simulink model "rectificador_pwm_para_ver_curvas_igbt"  (R2024a)
settings: Solver=ode23t  StartTime=0.0  StopTime=2  FixedStep=sim_sample_time  MaxStep=1e-5  RelTol=1e-9
undefined symbols (not defined in the file or in its folder): config, gcbh, sps_rtmsupport, spsTwoLevelConverterModel, SwitchingDevices
libraries: spsIGBTDiodeLib x6, slpidlib x3, spsSeriesRLCBranchLib x2, spsabctodq0Lib x2, simulink x2, spsThreePhaseVIMeasurementLib x2, spsDCVoltageSourceLib x1, spsGroundLib x1, spsPLL3phLib x1, spsSVPWMGenerator2LevelLib x1, spsdq0toAlphaBetaZeroLib x1, spsdq0toabcLib x1
settings Model: SimulationMode=accelerator  PauseTimes=0.05  Creator=sebar  LastModifiedBy=sebar
settings SolverCC: ZeroCrossAlgorithm=Adaptive  AlgebraicLoopSolver=TrustRegion  DecoupledContinuousIntegration=on  ODENIntegrationMethod=ode14x
settings DataIOCC: ExternalInput=getinputstruct(op_trim1)  InitialState=steady_state  LimitDataPoints=on  LoadInitialState=on  SaveFinalState=on  SaveFormat=Array  SaveOutput=off  SignalLogging=off  DSMLogging=off  SaveTime=off
settings OptimizationCC: LifeSpan=inf
settings DebuggingCC: ReadBeforeWriteMsg=DisableAll  WriteAfterWriteMsg=DisableAll  WriteAfterReadMsg=DisableAll  IgnoredZcDiagnostic=none  SolverPrmCheckMsg=warning  MultiTaskDSMMsg=none  SFUnexpectedBacktrackingDiag=warning  SFNoUnconditionalDefaultTransitionDiag=warning  SFExecutionAtInitializationDiag=none  ArithmeticOperatorsInVariantConditions=warning
settings HardwareCC: ProdBitPerPointer=32  ProdBitPerSizeT=32  ProdBitPerPtrDiffT=32  ProdLargestAtomicFloat=None  ProdIntDivRoundTo=Undefined  ProdEndianess=Unspecified  ProdWordSize=32  ProdHWDeviceType=32-bit Generic
settings ModelReferenceCC: UpdateModelReferenceTargets=IfOutOfDate  PropagateSignalLabelsOutOfModel=off
settings SFSimCC: SFSimEcho=off  SimUseLocalCustomCode=off  CustomCodeUndefinedFunction=UseInterfaceOnly  SimTargetLang=C++  GPUAcceleration=on  SimDLTargetLibrary=cudnn
settings RTWCC: RTWUseLocalCustomCode=off  GPUComputeCapability=3.5
settings CodeAppCC: StateflowObjectComments=on
settings GRTTargetCC: TargetLangStandard=C89/C90 (ANSI)
settings ConfigComp: CovMetricSettings=dw  CovSaveCumulativeToWorkspaceVar=on  CovSaveSingleToWorkspaceVar=on  CovExternalEMLEnable=off  CovSFcnEnable=off
settings SimscapeCC: SimscapeNormalizeSystem=off

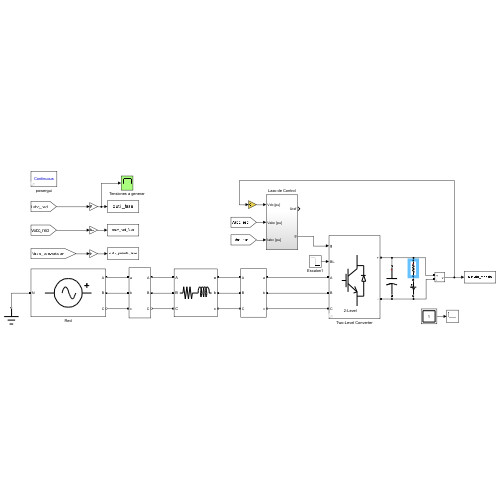
[thumbnail: Simulink's stored preview of the top-level diagram]
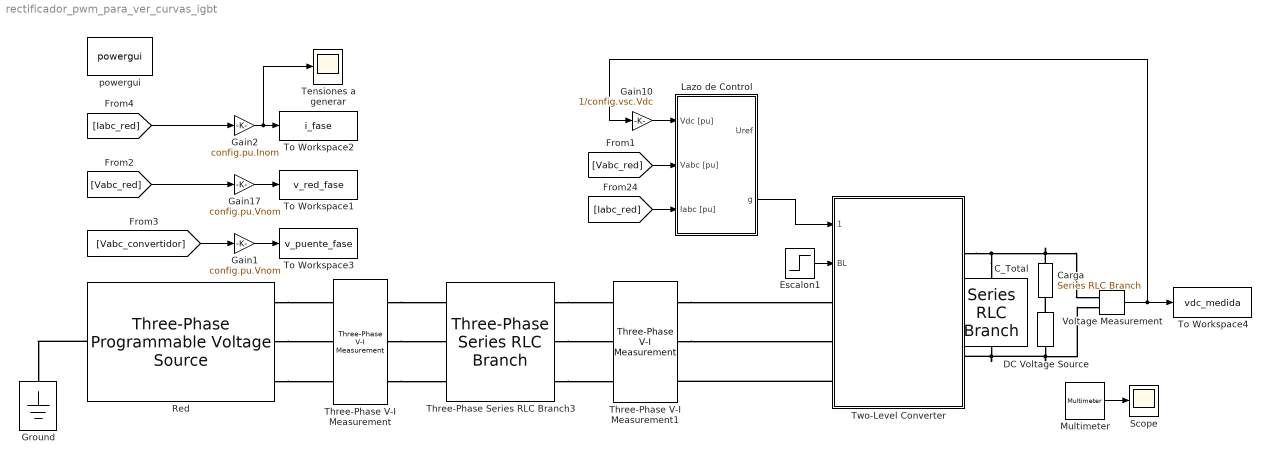
== system rectificador_pwm_para_ver_curvas_igbt ==
  C_Total : spsSeriesRLCBranchLib/Series RLC Branch  LConnTagsString=__new0  RConnTagsString=__new0  BranchType=C  Resistance=1  Inductance=1e-3  SetiL0=off  InitialCurrent=0  Capacitance=config.vsc.C  Setx0=on  InitialVoltage=config.vsc.Vdc  Measurements=Branch current
  Carga : spsSeriesRLCBranchLib/Series RLC Branch  LConnTagsString=__new0  RConnTagsString=__new0  BranchType=R  Resistance=config.vsc.R_load * ~config.usar_fuente_lado_DC + 1e-6 * config.usar_fuente_lado_DC  Inductance=1e-3  SetiL0=off  InitialCurrent=0  Capacitance=1e-6  Setx0=off  InitialVoltage=0  Measurements=None
  DC Voltage Source : spsDCVoltageSourceLib/DC Voltage Source  Amplitude=config.vsc.Vdc * config.usar_fuente_lado_DC  Measurements=None
  Escalon1 : Step  Time=0.25*(config.mode == ModoControl.SOLO_FEEDFORWARD)*0  Before=1  After=0  SampleTime=1e-5
  Gain1 : Gain  Gain=config.pu.Vnom
  Gain10 : Gain  Gain=1/config.vsc.Vdc
  Gain17 : Gain  Gain=config.pu.Vnom
  Gain2 : Gain  Gain=config.pu.Inom
  Ground : spsGroundLib/Ground  LConnTagsString=a
  Lazo de Control : Subsystem
  Multimeter : spsMultimeterLib/Multimeter  L=1  sel=1  yselected={}  Gain=1  OutputType=Complex  PlotAtSimulationStop=off  PhasorSimulation=off
  Red : spsThreePhaseProgrammableVoltageSourceLib/Three-Phase Programmable Voltage Source  PositiveSequence="[28*sqrt(3)  0 50]"  VariationEntity=None  VariationType=Step  VariationTypeAlt=Step  VariationStep=1  VariationRate=10  VariationMagnitude=0.3  VariationFrequency=2  VariationTiming=[1 2]  VariationPhaseA=off  Amplitudes=[1 0.8 1.2 1.0]  TimeValues=[0 0.1 0.15 0.2]  HarmonicGeneration=off  HarmonicA=[3 0.2 -25 0]  HarmonicB=[2 0.15 35 2]  Timing="[0.05  3]"  BusType=swing  Pref=0  Qref=0  Qmin=-inf  Qmax=inf
  Scope : Scope
  Tensiones a generar : Scope
  Three-Phase Series RLC Branch3 : spsThreePhaseSeriesRLCBranchLib/Three-Phase Series RLC Branch  LConnTagsString=A|B|C  RConnTagsString=A|B|C  BranchType=RL  Resistance=config.vsc.R  Inductance=config.vsc.L  Capacitance=1e-6  Measurements=None
  Three-Phase V-I Measurement : spsThreePhaseVIMeasurementLib/Three-Phase V-I Measurement  VoltageMeasurement=phase-to-ground  SetLabelV=on  LabelV=Vabc_red  Vpu=on  VpuLL=off  CurrentMeasurement=yes  SetLabelI=on  LabelI=Iabc_red  Ipu=on  Pbase=config.pu.Pnom  Vbase=config.pu.Vnom * sqrt(3) / sqrt(2)  OutputType=Complex  PhasorSimulation=off  PSBequivalent=0
  Three-Phase V-I Measurement1 : spsThreePhaseVIMeasurementLib/Three-Phase V-I Measurement  VoltageMeasurement=phase-to-ground  SetLabelV=on  LabelV=Vabc_convertidor  Vpu=on  VpuLL=off  CurrentMeasurement=no  SetLabelI=off  LabelI=Iabc  Ipu=off  Pbase=100e6  Vbase=config.pu.Vnom * sqrt(3) / sqrt(2)  OutputType=Complex  PhasorSimulation=off  PSBequivalent=0
  To Workspace1 : ToWorkspace  VariableName=v_red_fase  SaveFormat=Timeseries  SampleTime=config.to_workspace_sample_time
  To Workspace2 : ToWorkspace  VariableName=i_fase  SaveFormat=Timeseries  SampleTime=config.to_workspace_sample_time
  To Workspace3 : ToWorkspace  VariableName=v_puente_fase  SaveFormat=Timeseries  SampleTime=config.to_workspace_sample_time
  To Workspace4 : ToWorkspace  VariableName=vdc_medida  SaveFormat=Timeseries  SampleTime=config.to_workspace_sample_time
  Two-Level Converter : Subsystem  AncestorBlock=sps_lib/Power Electronics/Two-Level Converter  DialogController=POWERSYS.PowerSysDialog  LoadFcn=sps_rtmsupport('LoadFcn',gcbh);  StartFcn=sps_rtmsupport('StartFcn',gcbh);  StopFcn=sps_rtmsupport('StopFcn',gcbh);  mask(Two-Level Converter){ModelType=Switching devices, Ron=1e-6, Rs=config.vsc.snubber.Rs, Cs=config.vsc.snubber.Cs, Vforward=[0,0], Ron_Diode=1e-3, Rs_Diode=1e6, Cs_Diode=inf, Vf_Diode=1e-3, Rs_CurrentSource=inf, Ron_ACsource=1e-3}
      mask prompts: ModelType "Model type:"; Ron "Device on-state resistance (Ohms)"; Rs "Snubber resistance (Ohms)"; Cs "Snubber capacitance (F)"; Vforward "Forward voltages [Device Vf(V), Diode Vfd(V)]"; Ron_Diode "Diode on-state resistance (Ohms)"; Rs_Diode "Diode snubber resistance (Ohms)"; Cs_Diode "Diode snubber capacitance (F)"; Vf_Diode "Diode forward voltage (V)"; Rs_CurrentSource "DC side snubber resistance (Ohms)"; Ron_ACsource "AC side source resistance (Ohms)"
      mask help:
      | Implements a three-phase two-level power converter using the following modeling techniques:
      |
      | 1. Switching devices: The converter is modeled with IGBT/diode pairs controlled by firing pulses produced by a PWM generator.
      |
      | 2. Switching function: The converter is modeled by a switching function controlled by firing pulses produced by a PWM generator (0/1 signals) or by firing pulses averaged over a specified period (PWM averaging: signals between 0 and 1).
      |
      | 3. Average model (Uref-controlled): The converter is modeled using a switching-function model directly controlled by the reference voltage. A PWM generator is not required.
      |
      | 4. Average model (Uref-controlled, no rectifier mode): The converter is modeled using voltage sources directly controlled by the reference voltage. A PWM generator is not required, and the rectifier mode is not simulated.
      |
      | Technique 1 is the most accurate, while technique 4 yields to the fastest simulation. Technique 2 (with firing pulses averaged), as well as techniques 3 and 4 are well-suited for real-time simulation.
      mask init:
      | block=gcb;
      | [WantBlockChoice,Ts,BLK] = powericon('PowerConverterCback',block,Ron,Rs,Cs,Vforward,Ron_Diode,Rs_Diode,Cs_Diode,Vf_Diode,Rs_CurrentSource, Ron_ACsource);
      | powericon('SetInternalModels','set',block,WantBlockChoice);
      settings: LibrarySourceBlock=sps_lib/Power Electronics/Two-Level Converter  CopyFcn=sps_rtmsupport('CopyFcn',gcbh);  DeleteFcn=sps_rtmsupport('DeleteFcn',gcbh);  UndoDeleteFcn=sps_rtmsupport('UndoDeleteFcn',gcbh);  ModelCloseFcn=sps_rtmsupport('ModelCloseFcn',gcbh);  PreSaveFcn=sps_rtmsupport('PreSaveFcn',gcbh);  PostSaveFcn=sps_rtmsupport('PostSaveFcn',gcbh);  NameChangeFcn=sps_rtmsupport('NameChangeFcn',gcbh);  PreCopyFcn=sps_rtmsupport('PreCopyFcn',gcbh);  OpenFcn=sps_rtmsupport('OpenFcn',gcbh, [1]);  CloseFcn=sps_rtmsupport('CloseFcn',gcbh);  PreDeleteFcn=sps_rtmsupport('PreDeleteFcn',gcbh);
      mask Help: helpview(psbhelp);
      mask TypeOptions ModelType: Switching devices | Switching function | Average model (Uref-controlled) | Average model (No rectifier mode)
      mask Callback ModelType: powericon('PowerConverterCback',gcb);
      mask Display:
      | x1=0.05;
      | y1=0.20;
      | %
      | plot([0.5 0.5]+x1,[0.97,0.8]-y1)
      | plot([0.5 0.32]+x1,[0.80 0.71]-y1)
      | plot([0.32 0.32]+x1,[0.80 0.52]-y1)
      | plot([0.32 0.5]+x1,[0.62 0.52]-y1)
      | plot([0.5 0.5]+x1,[0.52 0.35]-y1)
      | plot([0.45 0.5 0.43]+x1,[0.59 0.52 0.51]-y1)
      | %
      | plot([0.28 0.28]+x1,[0.74 0.58]-y1)
      | plot([0.28 0.20]+x1,[0.66 0.66]-y1)
      | %
      | plot([0.5 0.63]+x1,[0.84 0.84]-y1)
      | plot([0.63 0.63]+x1,[0.84 0.72]-y1)
      | plot([0.63 0.59]+x1,[0.72 0.65]-y1)
      | plot([0.63 0.67]+x1,[0.72 0.65]-y1)
      | plot([0.59 0.67]+x1,[0.65 0.65]-y1)
      | plot([0.63 0.63]+x1,[0.65 0.47]-y1)
      | plot([0.5 0.63]+x1,[0.47 0.47]-y1)
      | plot([0.58 0.67]+x1,[0.72 0.72]-y1)
      | %
      | text(0.3,0.1,'2-Level')
      | if ModelType==3 |ModelType==4
      |    port_label('input',1,'Uref')
      | else
      |     port_label('input',1,'g')
      | end
  Voltage Measurement : spsVoltageMeasurementLib/Voltage Measurement  PhasorSimulation=off  OutputType=Complex  PSBequivalent=0
  powergui : sps_lib/powergui  Priority=1  SimulationMode=Continuous  SampleTime=config.sample_time  frequency=50  Iterations=50  frequencyindice=0  Pbase=100e6  ErrMax=1e-4  UnitsV=kV  UnitsW=MW  buscounter=0  FunctionMessages=off  echomessages=off  EnableUseOfTLC=off  CurrentSourceSwitches=on  DisableSnubberDevices=off  DisableRonSwitches=off  DisableVfSwitches=off  DisplayEquations=off  AutomaticDiscreteSolvers=off  SolverType=Tustin  Interpol=off  ExternalGateDelay=off  methode=on  Ts=100  x0status=blocks  SPID=off  SwTol=0  HookPort=off  NonlinearTolerance=1e-4  nMaxIteration=100  ContinueOnMaxIteration=off  RestoreLinks=warning  ResistiveCurrentMeasurement=off  Frange=[0:2:500]  Ylog=off  Xlog=on  ShowGrid=off  save=off  variable=ZData  structure=0  ZoomFFT=off  StartTime=0.0  cycles=1  DisplayStyle=1  fundamental=60  FreqAxis=off  MaxFrequency=1000  frequencyindicesteady=1  RmsSteady=1  display=off
  wires:
  Gain10/1 -> Lazo de Control/1(Vdc [pu])
  [Vabc_red] -> Lazo de Control/2(Vabc [pu])
  [Iabc_red] -> Lazo de Control/3(Iabc [pu])
  [Vabc_convertidor] -> Gain1/1
  [Vabc_red] -> Gain17/1
  Voltage Measurement/1 -> Gain10/1, To Workspace4/1
  Gain17/1 -> To Workspace1/1
  Gain1/1 -> To Workspace3/1
  Escalon1/1 -> Two-Level Converter/2(BL)
  Gain2/1 -> Tensiones a generar/1, To Workspace2/1
  [Iabc_red] -> Gain2/1
  Lazo de Control/2(g) -> Two-Level Converter/1("  ")
  Multimeter/1 -> Scope/1
  connections:
  Red/LConn1 -- Ground/LConn1
  C_Total/RConn1 -- DC Voltage Source/LConn1 -- Voltage Measurement/LConn2 -- Two-Level Converter/RConn2
  C_Total/LConn1 -- Carga/LConn1 -- Voltage Measurement/LConn1 -- Two-Level Converter/RConn1
  Three-Phase Series RLC Branch3/RConn1 -- Three-Phase V-I Measurement1/LConn1
  Three-Phase Series RLC Branch3/RConn2 -- Three-Phase V-I Measurement1/LConn2
  Three-Phase Series RLC Branch3/RConn3 -- Three-Phase V-I Measurement1/LConn3
  Three-Phase V-I Measurement1/RConn1 -- Two-Level Converter/LConn1
  Three-Phase V-I Measurement1/RConn2 -- Two-Level Converter/LConn2
  Two-Level Converter/LConn3 -- Three-Phase V-I Measurement1/RConn3
  Three-Phase V-I Measurement/LConn1 -- Three-Phase Series RLC Branch3/LConn1
  Three-Phase V-I Measurement/LConn2 -- Three-Phase Series RLC Branch3/LConn2
  Three-Phase V-I Measurement/LConn3 -- Three-Phase Series RLC Branch3/LConn3
  Red/RConn1 -- Three-Phase V-I Measurement/RConn1
  Red/RConn2 -- Three-Phase V-I Measurement/RConn2
  Red/RConn3 -- Three-Phase V-I Measurement/RConn3
  DC Voltage Source/RConn1 -- Carga/RConn1

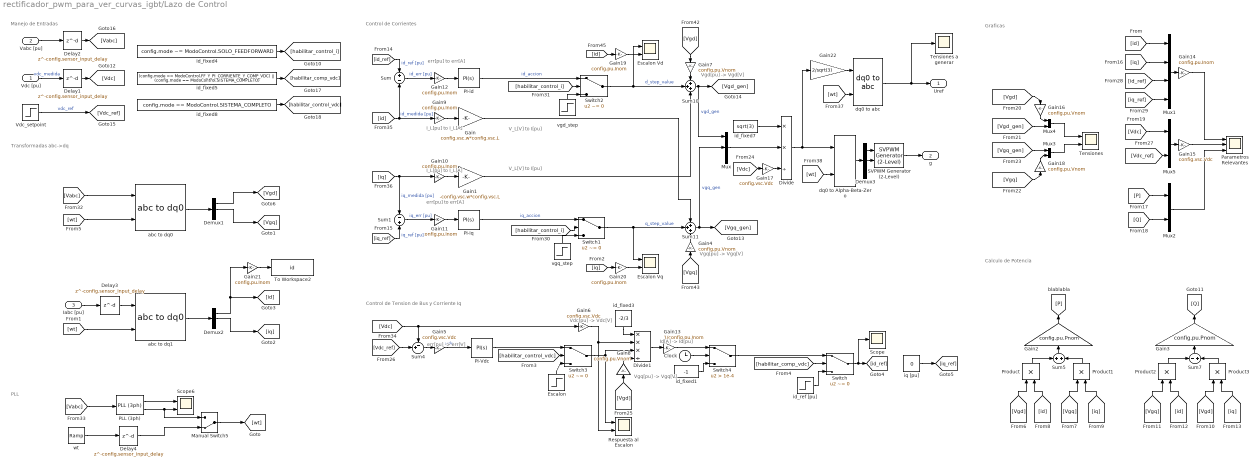
== system rectificador_pwm_para_ver_curvas_igbt/Lazo de Control ==
  note: Transformadas abc->dq
  note: I_L[pu] to I_L[A]
  note: Calculo de Potencia
  note: Graficas
  note: PLL
  note: Manejo de Entradas
  note: Control de Tension de Bus y Corriente Iq
  note: Control de Corrientes
  note: V_L[V] to I[pu]
  note: Vgd[pu] -> Vgd[V]
  note: I_L[pu] to I_L[A]
  note: Vgq[pu] -> Vgq[V]
  note: Vgq[pu] -> Vgq[V]
  note: Id[A] -> Id[pu]
  note: err[pu] -> err[V]
  note: err[pu] to err[A]
  note: err[pu] to err[A]
  note: Vdc[pu] -> Vdc[V]
  note: V_L[V] to I[pu]
  Vdc [pu] : Inport
  Vabc [pu] : Inport  Port=2
  Iabc [pu] : Inport  Port=3
  Clock : Clock
  Delay1 : Delay  DelayLength=config.sensor_input_delay  InitialCondition=1  SampleTime=config.sensor_input_sample_time
  Delay2 : Delay  DelayLength=config.sensor_input_delay  InitialCondition=1  SampleTime=config.sensor_input_sample_time
  Delay3 : Delay  DelayLength=config.sensor_input_delay  InitialCondition=1  SampleTime=config.sensor_input_sample_time
  Delay4 : Delay  DelayLength=config.sensor_input_delay  InitialCondition=0  SampleTime=config.sensor_input_sample_time
  Demux1 : Demux  Outputs=3
  Demux2 : Demux  Outputs=3
  Demux3 : Demux  Outputs=3
  Divide : Product  Inputs=**/
  Divide1 : Product  Inputs=***/
  Escalon : Step  Time=config.step.id.time  Before=config.step.id.start_value  After=config.step.id.end_value  SampleTime=1e-5
  Escalon Vd : Scope  NumInputPorts=2
  Escalon Vq : Scope  NumInputPorts=2
  Gain : Gain  Gain=config.vsc.w*config.vsc.L
  Gain1 : Gain  Gain=-config.vsc.w*config.vsc.L
  Gain{9..12,14,19..21} (8 alike) : Gain  Gain=config.pu.Inom
  Gain13 : Gain  Gain=1/config.pu.Inom
  Gain{5..6,15,17} (4 alike) : Gain  Gain=config.vsc.Vdc
  Gain{4,7..8,16,18} (5 alike) : Gain  Gain=config.pu.Vnom
  Gain2 : Gain  Gain=config.pu.Pnom
  Gain22 : Gain  Gain=2/sqrt(3)
  Gain3 : Gain  Gain=config.pu.Pnom
  Manual Switch5 : ManualSwitch  CurrentSetting=0
  Mux : Mux  Inputs=3
  Mux1 : Mux
  Mux{2..5} (4 alike) : Mux  Inputs=2
  PI-Vdc : slpidlib/PID Controller  Controller=PI  Form=Parallel  TimeDomain=Continuous-time  UseExternalTs=off  SampleTime=1  IntegratorMethod=Forward Euler  FilterMethod=Forward Euler  ControllerParametersSource=internal  P=config.ContDC.Kp  I=config.ContDC.Ki  UseKiTs=off  D=0  UseExternalDerivativeSource=off  N=100  UseFilter=on  TunerSelectOption=Transfer Function Based (PID Tuner App)  InitialConditionSource=internal  InitialConditionForIntegrator=0  InitialConditionForFilter=0  DifferentiatorICPrevScaledInput=0  ExternalReset=none  TrackingMode=off  Kt=1  LimitOutput=off  SatLimitsSource=internal  UpperSaturationLimit=inf  LowerSaturationLimit=-inf  LinearizeAsGain=on  AntiWindupMode=none  Kb=1  LimitIntegrator=off  UpperIntegratorSaturationLimit=inf  LowerIntegratorSaturationLimit=-inf  POutMin=[]  POutMax=[]  IOutMin=[]  IOutMax=[]  DOutMin=[]  DOutMax=[]  NOutMin=[]  NOutMax=[]  SumOutMin=[]  SumOutMax=[]  SaturationOutMin=[]  SaturationOutMax=[]  PParamMin=[]  PParamMax=[]  IParamMin=[]  IParamMax=[]  DParamMin=[]  DParamMax=[]  NParamMin=[]  NParamMax=[]  KbParamMin=[]  KbParamMax=[]  KtParamMin=[]  KtParamMax=[]  KbOutMin=[]  KbOutMax=[]  KtOutMin=[]  KtOutMax=[]  IntegratorOutMin=[]  IntegratorOutMax=[]  FilterOutMin=[]  FilterOutMax=[]  SumI1OutMin=[]  SumI1OutMax=[]  SumI2OutMin=[]  SumI2OutMax=[]  SumI3OutMin=[]  SumI3OutMax=[]  SumI4OutMin=[]  SumI4OutMax=[]  SumDOutMin=[]  SumDOutMax=[]  DifferentiatorOutMin=[]  DifferentiatorOutMax=[]  FilterDiffOutCoefMin=[]  FilterDiffOutCoefMax=[]  ReciprocalOutMin=[]  ReciprocalOutMax=[]  SumDenOutMin=[]  SumDenOutMax=[]  SumNumOutMin=[]  SumNumOutMax=[]  DivideOutMin=[]  DivideOutMax=[]  UdiffTsProdOutMin=[]  UdiffTsProdOutMax=[]  NTsProdOutMin=[]  NTsProdOutMax=[]  UintegralTsProdOutMin=[]  UintegralTsProdOutMax=[]  UngainTsProdOutMin=[]  UngainTsProdOutMax=[]  ClampingZeroOutDataTypeStr=Inherit: Inherit via back propagation  ClampingZeroOutMin=[]  ClampingZeroOutMax=[]  FilterDenConstantOutDataTypeStr=Inherit: Inherit via back propagation  FilterDenConstantOutMin=[]  FilterDenConstantOutMax=[]  PCopyOutDataTypeStr=Inherit: Inherit via back propagation  PCopyOutMin=[]  PCopyOutMax=[]  NCopyOutDataTypeStr=Inherit: Inherit via back propagation  NCopyOutMin=[]  NCopyOutMax=[]  IntegratorContinuousStateAttributes=''  IntegratorStateMustResolveToSignalObject=off  IntegratorRTWStateStorageClass=Auto  FilterContinuousStateAttributes=''  FilterStateMustResolveToSignalObject=off  FilterRTWStateStorageClass=Auto  ParallelPVariant=InternalParameters  IdealPVariant=Disabled  IVariant=InternalParameters  DVariant=Disabled  IntegratorVariant=Continuous  SatVariant=Disabled  AWVariant=Passthrough  PCopyVariant=Disabled  TRVariant=Disabled  FdbkBlocksVariant=Forward  IdealPFdbkVariant=Disabled  SatFdbkVariant=Disabled  DerivativeFilterVariant=Disabled  NVariant=Disabled  NCopyVariant=Disabled_SignalSpec  FilterICVariant=Disabled  IntegratorICVariant=InternalICs  ExternalResetVariant=Disabled  TRSumVariant=Passthrough  SumFdbkVariant=Disabled  SumVariant=Sum_PI  TsampFilterVariant=InternalTs  TsampNgainVariant=Passthrough  TsampIntegralVariant=Disabled_SignalSpec  ExternalSaturationOutDataTypeStr=Inherit: Same as second input  DerivativeSourceVariant=Disabled
  PI-id : slpidlib/PID Controller  Controller=PI  Form=Parallel  TimeDomain=Continuous-time  UseExternalTs=off  SampleTime=1  IntegratorMethod=Forward Euler  FilterMethod=Forward Euler  ControllerParametersSource=internal  P=config.ContI.Kp  I=config.ContI.Ki  UseKiTs=off  D=0  UseExternalDerivativeSource=off  N=100  UseFilter=on  TunerSelectOption=Transfer Function Based (PID Tuner App)  InitialConditionSource=internal  InitialConditionForIntegrator=0  InitialConditionForFilter=0  DifferentiatorICPrevScaledInput=0  ExternalReset=none  TrackingMode=off  Kt=1  LimitOutput=off  SatLimitsSource=internal  UpperSaturationLimit=20  LowerSaturationLimit=-20  LinearizeAsGain=on  AntiWindupMode=none  Kb=1  LimitIntegrator=off  UpperIntegratorSaturationLimit=inf  LowerIntegratorSaturationLimit=-inf  POutMin=[]  POutMax=[]  IOutMin=[]  IOutMax=[]  DOutMin=[]  DOutMax=[]  NOutMin=[]  NOutMax=[]  SumOutMin=[]  SumOutMax=[]  SaturationOutMin=[]  SaturationOutMax=[]  PParamMin=[]  PParamMax=[]  IParamMin=[]  IParamMax=[]  DParamMin=[]  DParamMax=[]  NParamMin=[]  NParamMax=[]  KbParamMin=[]  KbParamMax=[]  KtParamMin=[]  KtParamMax=[]  KbOutMin=[]  KbOutMax=[]  KtOutMin=[]  KtOutMax=[]  IntegratorOutMin=[]  IntegratorOutMax=[]  FilterOutMin=[]  FilterOutMax=[]  SumI1OutMin=[]  SumI1OutMax=[]  SumI2OutMin=[]  SumI2OutMax=[]  SumI3OutMin=[]  SumI3OutMax=[]  SumI4OutMin=[]  SumI4OutMax=[]  SumDOutMin=[]  SumDOutMax=[]  DifferentiatorOutMin=[]  DifferentiatorOutMax=[]  FilterDiffOutCoefMin=[]  FilterDiffOutCoefMax=[]  ReciprocalOutMin=[]  ReciprocalOutMax=[]  SumDenOutMin=[]  SumDenOutMax=[]  SumNumOutMin=[]  SumNumOutMax=[]  DivideOutMin=[]  DivideOutMax=[]  UdiffTsProdOutMin=[]  UdiffTsProdOutMax=[]  NTsProdOutMin=[]  NTsProdOutMax=[]  UintegralTsProdOutMin=[]  UintegralTsProdOutMax=[]  UngainTsProdOutMin=[]  UngainTsProdOutMax=[]  ClampingZeroOutDataTypeStr=Inherit: Inherit via back propagation  ClampingZeroOutMin=[]  ClampingZeroOutMax=[]  FilterDenConstantOutDataTypeStr=Inherit: Inherit via back propagation  FilterDenConstantOutMin=[]  FilterDenConstantOutMax=[]  PCopyOutDataTypeStr=Inherit: Inherit via back propagation  PCopyOutMin=[]  PCopyOutMax=[]  NCopyOutDataTypeStr=Inherit: Inherit via back propagation  NCopyOutMin=[]  NCopyOutMax=[]  IntegratorContinuousStateAttributes=''  IntegratorStateMustResolveToSignalObject=off  IntegratorRTWStateStorageClass=Auto  FilterContinuousStateAttributes=''  FilterStateMustResolveToSignalObject=off  FilterRTWStateStorageClass=Auto  ParallelPVariant=InternalParameters  IdealPVariant=Disabled  IVariant=InternalParameters  DVariant=Disabled  IntegratorVariant=Continuous  SatVariant=Disabled  AWVariant=Passthrough  PCopyVariant=Disabled  TRVariant=Disabled  FdbkBlocksVariant=Forward  IdealPFdbkVariant=Disabled  SatFdbkVariant=Disabled  DerivativeFilterVariant=Disabled  NVariant=Disabled  NCopyVariant=Disabled_SignalSpec  FilterICVariant=Disabled  IntegratorICVariant=InternalICs  ExternalResetVariant=Disabled  TRSumVariant=Passthrough  SumFdbkVariant=Disabled  SumVariant=Sum_PI  TsampFilterVariant=InternalTs  TsampNgainVariant=Passthrough  TsampIntegralVariant=Disabled_SignalSpec  ExternalSaturationOutDataTypeStr=Inherit: Same as second input  DerivativeSourceVariant=Disabled
  PI-iq : slpidlib/PID Controller  Controller=PI  Form=Parallel  TimeDomain=Continuous-time  UseExternalTs=off  SampleTime=1  IntegratorMethod=Forward Euler  FilterMethod=Forward Euler  ControllerParametersSource=internal  P=config.ContI.Kp  I=config.ContI.Ki  UseKiTs=off  D=0  UseExternalDerivativeSource=off  N=100  UseFilter=on  TunerSelectOption=Transfer Function Based (PID Tuner App)  InitialConditionSource=internal  InitialConditionForIntegrator=0  InitialConditionForFilter=0  DifferentiatorICPrevScaledInput=0  ExternalReset=none  TrackingMode=off  Kt=1  LimitOutput=off  SatLimitsSource=internal  UpperSaturationLimit=20  LowerSaturationLimit=-20  LinearizeAsGain=on  AntiWindupMode=none  Kb=1  LimitIntegrator=off  UpperIntegratorSaturationLimit=inf  LowerIntegratorSaturationLimit=-inf  POutMin=[]  POutMax=[]  IOutMin=[]  IOutMax=[]  DOutMin=[]  DOutMax=[]  NOutMin=[]  NOutMax=[]  SumOutMin=[]  SumOutMax=[]  SaturationOutMin=[]  SaturationOutMax=[]  PParamMin=[]  PParamMax=[]  IParamMin=[]  IParamMax=[]  DParamMin=[]  DParamMax=[]  NParamMin=[]  NParamMax=[]  KbParamMin=[]  KbParamMax=[]  KtParamMin=[]  KtParamMax=[]  KbOutMin=[]  KbOutMax=[]  KtOutMin=[]  KtOutMax=[]  IntegratorOutMin=[]  IntegratorOutMax=[]  FilterOutMin=[]  FilterOutMax=[]  SumI1OutMin=[]  SumI1OutMax=[]  SumI2OutMin=[]  SumI2OutMax=[]  SumI3OutMin=[]  SumI3OutMax=[]  SumI4OutMin=[]  SumI4OutMax=[]  SumDOutMin=[]  SumDOutMax=[]  DifferentiatorOutMin=[]  DifferentiatorOutMax=[]  FilterDiffOutCoefMin=[]  FilterDiffOutCoefMax=[]  ReciprocalOutMin=[]  ReciprocalOutMax=[]  SumDenOutMin=[]  SumDenOutMax=[]  SumNumOutMin=[]  SumNumOutMax=[]  DivideOutMin=[]  DivideOutMax=[]  UdiffTsProdOutMin=[]  UdiffTsProdOutMax=[]  NTsProdOutMin=[]  NTsProdOutMax=[]  UintegralTsProdOutMin=[]  UintegralTsProdOutMax=[]  UngainTsProdOutMin=[]  UngainTsProdOutMax=[]  ClampingZeroOutDataTypeStr=Inherit: Inherit via back propagation  ClampingZeroOutMin=[]  ClampingZeroOutMax=[]  FilterDenConstantOutDataTypeStr=Inherit: Inherit via back propagation  FilterDenConstantOutMin=[]  FilterDenConstantOutMax=[]  PCopyOutDataTypeStr=Inherit: Inherit via back propagation  PCopyOutMin=[]  PCopyOutMax=[]  NCopyOutDataTypeStr=Inherit: Inherit via back propagation  NCopyOutMin=[]  NCopyOutMax=[]  IntegratorContinuousStateAttributes=''  IntegratorStateMustResolveToSignalObject=off  IntegratorRTWStateStorageClass=Auto  FilterContinuousStateAttributes=''  FilterStateMustResolveToSignalObject=off  FilterRTWStateStorageClass=Auto  ParallelPVariant=InternalParameters  IdealPVariant=Disabled  IVariant=InternalParameters  DVariant=Disabled  IntegratorVariant=Continuous  SatVariant=Disabled  AWVariant=Passthrough  PCopyVariant=Disabled  TRVariant=Disabled  FdbkBlocksVariant=Forward  IdealPFdbkVariant=Disabled  SatFdbkVariant=Disabled  DerivativeFilterVariant=Disabled  NVariant=Disabled  NCopyVariant=Disabled_SignalSpec  FilterICVariant=Disabled  IntegratorICVariant=InternalICs  ExternalResetVariant=Disabled  TRSumVariant=Passthrough  SumFdbkVariant=Disabled  SumVariant=Sum_PI  TsampFilterVariant=InternalTs  TsampNgainVariant=Passthrough  TsampIntegralVariant=Disabled_SignalSpec  ExternalSaturationOutDataTypeStr=Inherit: Same as second input  DerivativeSourceVariant=Disabled
  PLL (3ph) : spsPLL3phLib/PLL (3ph)  Fmin=45  Par_Init=[0, config.vsc.f]  ParK=[180, 3200, 1]  TcD=1e-4  MaxRateChangeFreq=12  FilterCutOffFreq=25  Ts=1 / config.vsc.f_sw  AGC=on
  Parametros Relevantes : Scope  NumInputPorts=3
  Product{,1..3} (4 alike) : Product
  Respuesta al Escalon : Scope  NumInputPorts=2
  SVPWM Generator (2-Level) : spsSVPWMGenerator2LevelLib/SVPWM Generator (2-Level)  InputType=alpha-beta components  SwitchingPattern=Pattern #1  Fc=config.vsc.f_sw  ParUref=[0.8 -30 50]  Ts=1/config.vsc.f_sw*0
  Scope : Scope
  Scope6 : Scope  NumInputPorts=2
  Sum : Sum  Inputs=+|-
  Sum1 : Sum  Inputs=-|+
  Sum10 : Sum  Inputs=+++
  Sum11 : Sum  Inputs=+++
  Sum4 : Sum  Inputs=-+|
  Sum5 : Sum  Inputs=+|+
  Sum7 : Sum  Inputs=-|+
  Switch{,1..3} (4 alike) : Switch  Criteria=u2 ~= 0  SaturateOnIntegerOverflow=off  InputSameDT=off
  Switch4 : Switch  Criteria=u2 > Threshold  Threshold=1e-4  SaturateOnIntegerOverflow=off  InputSameDT=off
  Tensiones : Scope  NumInputPorts=2
  Tensiones a generar : Scope
  To Workspace2 : ToWorkspace  VariableName=id  SaveFormat=Timeseries  SampleTime=config.to_workspace_sample_time
  Vdc_setpoint : Step  Time=(~config.cambio_tension_referencia)*100000 + 2  Before=1  After=1 * (1 + config.step_setpoint_tension/100)  SampleTime=0
  abc to dq0 : spsabctodq0Lib/abc to dq0  Alignment=90 degrees behind phase A axis
  abc to dq1 : spsabctodq0Lib/abc to dq0  Alignment=90 degrees behind phase A axis
  dq0 to Alpha-Beta-Zero : spsdq0toAlphaBetaZeroLib/dq0 to Alpha-Beta-Zero  Alignment=90 degrees behind phase A axis
  dq0 to abc : spsdq0toabcLib/dq0 to abc  Alignment=90 degrees behind phase A axis
  id_fixed1 : Constant  Value=-1
  id_fixed3 : Constant  Value=-2/3
  id_fixed4 : Constant  Value=config.mode ~= ModoControl.SOLO_FEEDFORWARD
  id_fixed5 : Constant  Value=(config.mode == ModoControl.FF_Y_PI_CORRIENTE_Y_COMP_VDC) || (config.mode == ModoControl.SISTEMA_COMPLETO)
  id_fixed7 : Constant  Value=sqrt(3)
  id_fixed8 : Constant  Value=config.mode == ModoControl.SISTEMA_COMPLETO
  id_ref [pu] : Step  Time=1.25  Before=-3.0707/config.pu.Inom  After=-3.0707/config.pu.Inom*(1 + config.step_setpoint_corriente/100)  SampleTime=0
  iq [pu] : Constant  Value=0
  vgd_step : Step  Time=config.step.vgd.time  Before=config.step.vgd.start_value  After=config.step.vgd.end_value  SampleTime=1e-5
  vgq_step : Step  Time=config.step.vgq.time  Before=config.step.vgq.start_value  After=config.step.vgq.end_value  SampleTime=1e-5
  wt : simulink/Sources/Ramp  slope=2*pi*50  start=0  InitialOutput=0
  Uref : Outport
  g : Outport  Port=2
  wires:
  [wt] -> abc to dq0/2
  Vabc [pu]/1 -> Delay2/1
  [wt] -> abc to dq1/2
  Iabc [pu]/1 -> Delay3/1
  abc to dq0/1 -> Demux1/1
  Demux1/1 -> [Vgd]
  Demux1/2 -> [Vgq]
  abc to dq1/1 -> Demux2/1
  [id] -> Gain9/1, Sum/2  "id_medida [pu]"
  [iq] -> Gain10/1, Sum1/1  "iq_medida [pu]"
  [id_ref] -> Sum/1  "id_ref [pu]"
  [iq_ref] -> Sum1/2  "iq_ref [pu]"
  Sum/1 -> Gain12/1  "id_err [pu]"
  Sum1/1 -> Gain11/1  "iq_err [pu]"
  PI-iq/1 -> Switch1/1  "iq_accion"
  Sum11/1 -> Mux/2, [Vgq_gen]  "vgq_gen"
  Vdc [pu]/1 -> Delay1/1  "vdc_medida"
  [Vdc_ref] -> Sum4/2
  Gain5/1 -> PI-Vdc/1  "vdc_err"
  Divide1/1 -> Gain13/1
  id_ref [pu]/1 -> Switch/3
  iq [pu]/1 -> [iq_ref]
  [P] -> Mux2/1
  [Q] -> Mux2/2
  [iq] -> Mux1/2
  [id] -> Mux1/1
  [Vdc] -> Mux5/1
  Mux1/1 -> Gain14/1
  Mux2/1 -> Parametros Relevantes/3
  [Vgd_gen] -> Mux4/2
  [Vgq_gen] -> Mux3/1
  Manual Switch5/1 -> [wt]
  PLL (3ph)/2 -> Scope6/2, Manual Switch5/1
  wt/1 -> Delay4/1
  PLL (3ph)/1 -> Scope6/1
  Gain17/1 -> Divide/3
  Switch3/1 -> Divide1/3, Respuesta al Escalon/1
  [Vgd] -> Gain8/1
  Mux/1 -> Divide/2
  Mux5/1 -> Gain15/1
  [Vdc_ref] -> Mux5/2
  [id_ref] -> Mux1/3
  [iq_ref] -> Mux1/4
  [habilitar_control_i] -> Switch1/2
  [habilitar_control_i] -> Switch2/2
  PI-id/1 -> Switch2/1  "id_accion"
  [Vabc] -> abc to dq0/1
  [Vabc] -> PLL (3ph)/1
  [Vdc] -> Gain6/1, Sum4/1
  Demux2/1 -> Gain21/1, [id]
  Demux2/2 -> [iq]
  Sum10/1 -> Mux/1, [Vgd_gen]  "vgd_gen"
  vgd_step/1 -> Switch2/3
  vgq_step/1 -> Switch1/3
  Switch2/1 -> Sum10/2, Escalon Vd/1  "d_step_value"
  [Vgd] -> Gain7/1
  Switch1/1 -> Sum11/2, Escalon Vq/1  "q_step_value"
  id_fixed3/1 -> Divide1/1
  id_fixed7/1 -> Divide/1
  [id] -> Gain19/1
  PI-Vdc/1 -> Switch3/1
  [habilitar_control_vdc] -> Switch3/2
  Escalon/1 -> Switch3/3
  [Vgq] -> Product1/1
  [Vgd] -> Product3/1
  [id] -> Product2/2
  Product1/1 -> Sum5/2
  Sum5/1 -> Gain2/1
  Sum7/1 -> Gain3/1
  Gain3/1 -> [Q]
  [id] -> Product/2
  [Vgd] -> Product/1
  Product3/1 -> Sum7/2
  Product/1 -> Sum5/1
  [iq] -> Product3/2
  [Vgq] -> Product2/1
  Gain2/1 -> [P]
  [iq] -> Product1/2
  Product2/1 -> Sum7/1
  Vdc_setpoint/1 -> [Vdc_ref]  "vdc_ref"
  [iq] -> Gain20/1
  Gain/1 -> Sum11/1
  Gain1/1 -> Sum10/3
  Gain8/1 -> Divide1/4
  Gain10/1 -> Gain1/1
  Gain9/1 -> Gain/1
  Gain12/1 -> PI-id/1
  Gain11/1 -> PI-iq/1
  Gain7/1 -> Sum10/1
  [Vgq] -> Gain4/1
  Gain4/1 -> Sum11/3
  Gain13/1 -> Switch4/1
  Sum4/1 -> Gain5/1
  Gain14/1 -> Parametros Relevantes/1
  Gain15/1 -> Parametros Relevantes/2
  [Vgd] -> Gain16/1
  [Vgq] -> Gain18/1
  Mux4/1 -> Tensiones/1
  Mux3/1 -> Tensiones/2
  Gain16/1 -> Mux4/1
  Gain18/1 -> Mux3/2
  [Vdc] -> Gain17/1
  Gain19/1 -> Escalon Vd/2
  Gain20/1 -> Escalon Vq/2
  [wt] -> dq0 to abc/2
  Delay1/1 -> [Vdc]
  Delay2/1 -> [Vabc]
  Delay3/1 -> abc to dq1/1
  Divide/1 -> dq0 to Alpha-Beta-Zero/1, Gain22/1
  dq0 to abc/1 -> Uref/1, Tensiones a generar/1
  Switch4/1 -> Switch/1
  id_fixed1/1 -> Switch4/3
  Clock/1 -> Switch4/2
  Gain6/1 -> Divide1/2, Respuesta al Escalon/2
  Delay4/1 -> Manual Switch5/2
  Gain21/1 -> To Workspace2/1
  id_fixed4/1 -> [habilitar_control_i]
  [habilitar_comp_vdc] -> Switch/2
  Switch/1 -> Scope/1, [id_ref]
  id_fixed5/1 -> [habilitar_comp_vdc]
  id_fixed8/1 -> [habilitar_control_vdc]
  Gain22/1 -> dq0 to abc/1
  [wt] -> dq0 to Alpha-Beta-Zero/2
  dq0 to Alpha-Beta-Zero/1 -> Demux3/1
  Demux3/1 -> SVPWM Generator (2-Level)/1
  Demux3/2 -> SVPWM Generator (2-Level)/2
  SVPWM Generator (2-Level)/1 -> g/1

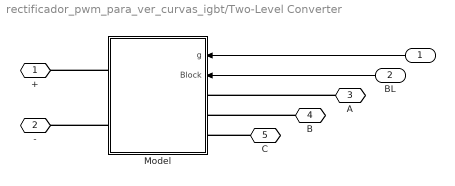
== system rectificador_pwm_para_ver_curvas_igbt/Two-Level Converter ==
  "  " : Inport
  BL : Inport  Port=2
  Model : Subsystem  AncestorBlock=spsTwoLevelConverterModel/SwitchingDevices
  + : PMIOPort  Side=Right
  - : PMIOPort  Port=2  Side=Right
  A : PMIOPort  Port=3  Side=Left
  B : PMIOPort  Port=4  Side=Left
  C : PMIOPort  Port=5  Side=Left
  wires:
  "  "/1 -> Model/1(g)
  BL/1 -> Model/2(Block)
  connections:
  C/RConn1 -- Model/LConn3
  B/RConn1 -- Model/LConn2
  A/RConn1 -- Model/LConn1
  Model/RConn2 -- -/RConn1
  Model/RConn1 -- +/RConn1

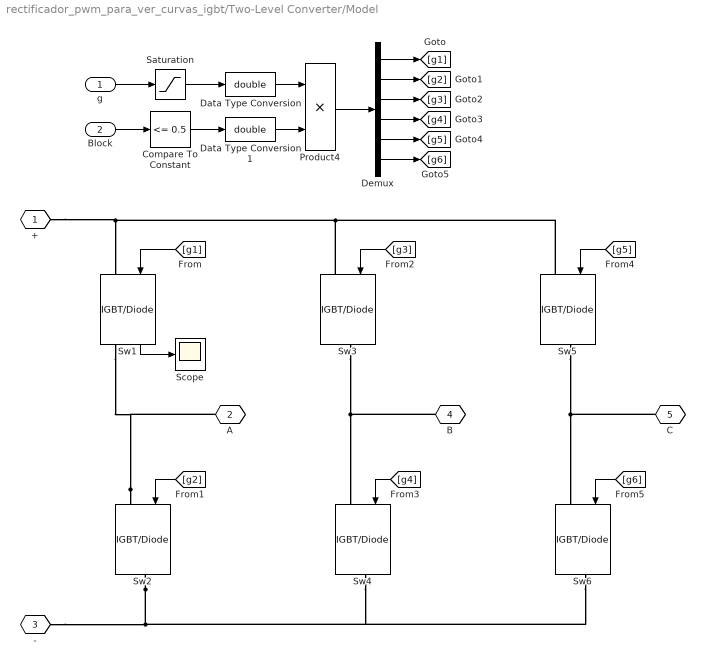
== system rectificador_pwm_para_ver_curvas_igbt/Two-Level Converter/Model ==
  g : Inport  PortDimensions=6
  Block : Inport  Port=2  PortDimensions=1
  Compare To Constant : simulink/Logic and Bit Operations/Compare To Constant  relop=<=  const=0.5  OutDataTypeStr=boolean
  Data Type Conversion : DataTypeConversion  OutDataTypeStr=double  SaturateOnIntegerOverflow=off  RndMeth=Floor
  Data Type Conversion1 : DataTypeConversion  OutDataTypeStr=double  SaturateOnIntegerOverflow=off  RndMeth=Floor
  Demux : Demux  Outputs=6
  Product4 : Product
  Saturation : Saturate  UpperLimit=1  LowerLimit=0
  Scope : Scope
  Sw1 : spsIGBTDiodeLib/IGBT//Diode  Ron=BLK.Ron  Rs=BLK.Rs  Cs=BLK.Cs  Measurements=on
  Sw{2..6} (5 alike) : spsIGBTDiodeLib/IGBT//Diode  Ron=BLK.Ron  Rs=BLK.Rs  Cs=BLK.Cs  Measurements=off
  + : PMIOPort  Tag=PMCPort  Side=Right
  A : PMIOPort  Tag=PMCPort  Port=2  Side=Left
  - : PMIOPort  Tag=PMCPort  Port=3  Side=Right
  B : PMIOPort  Tag=PMCPort  Port=4  Side=Left
  C : PMIOPort  Tag=PMCPort  Port=5  Side=Left
  wires:
  [g6] -> Sw6/1
  [g4] -> Sw4/1
  [g2] -> Sw2/1
  [g5] -> Sw5/1
  [g3] -> Sw3/1
  [g1] -> Sw1/1
  Demux/6 -> [g6]
  Demux/5 -> [g5]
  Demux/4 -> [g4]
  Demux/3 -> [g3]
  Demux/2 -> [g2]
  Demux/1 -> [g1]
  Saturation/1 -> Data Type Conversion/1
  Product4/1 -> Demux/1
  Block/1 -> Compare To Constant/1
  Compare To Constant/1 -> Data Type Conversion1/1
  Data Type Conversion1/1 -> Product4/2
  Data Type Conversion/1 -> Product4/1
  g/1 -> Saturation/1
  Sw1/1 -> Scope/1
  connections:
  C/RConn1 -- Sw5/RConn1 -- Sw6/LConn1
  B/RConn1 -- Sw4/LConn1 -- Sw3/RConn1
  Sw2/RConn1 -- Sw4/RConn1 -- Sw6/RConn1 -- -/RConn1
  Sw3/LConn1 -- Sw5/LConn1 -- Sw1/LConn1 -- +/RConn1
  Sw2/LConn1 -- A/RConn1 -- Sw1/RConn1
